simulink model "dualFisheyeSim"  (R2024b)
settings: Solver=VariableStepAuto  StartTime=0.0  StopTime=10.0  RelTol=1e-3
undefined symbols (not defined in the file): Sim3dSensor
libraries: sim3dcameralib x2, sim3dautolib x1, sim3dlib x1, visionsinks x1
settings Model: Creator=cuixingxing  LastModifiedBy=Administrator
settings ModelReferenceCC: EnableRefExpFcnMdlSchedulingChecks=on
settings RTWCC: GPUComputeCapability=3.5

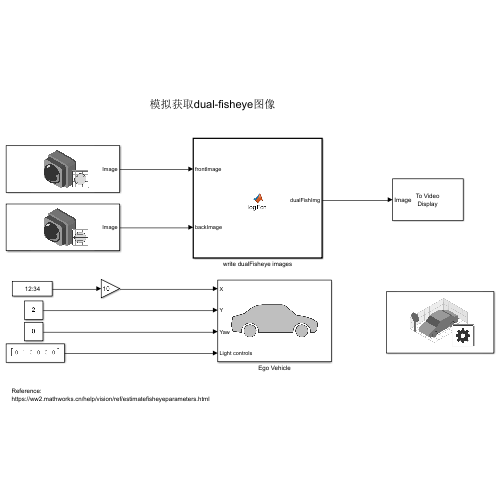
[thumbnail: Simulink's stored preview of the top-level diagram]
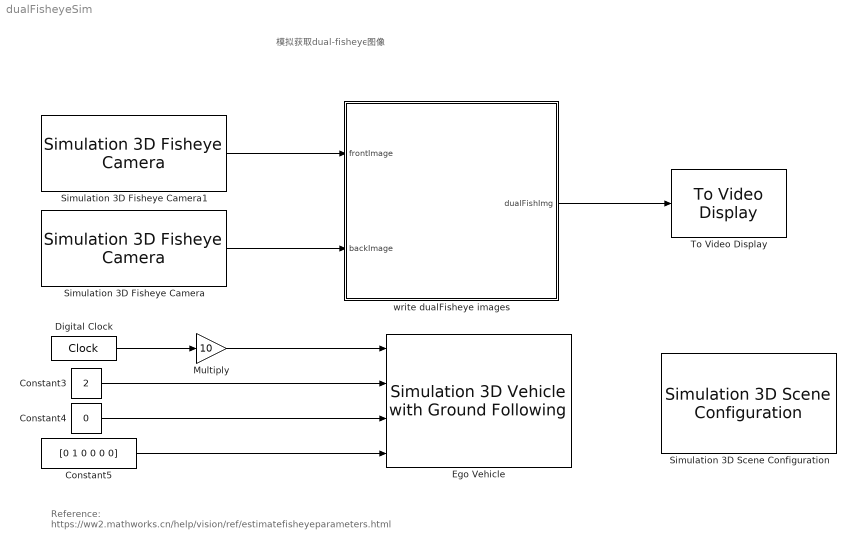
== system dualFisheyeSim ==
  note: Reference:
      | https://ww2.mathworks.cn/help/vision/ref/estimatefisheyeparameters.html
  note: 模拟获取dual-fisheye图像
  Constant3 : Constant  Value=2
  Constant4 : Constant  Value=0
  Constant5 : Constant  Value=[0 1 0 0 0 0]
  Digital Clock : DigitalClock  SampleTime=0.01
  Ego Vehicle : sim3dautolib/Simulation 3D Vehicle with Ground Following  Priority=-1  PassVehMesh=Hatchback  MeshPath=/MathWorksSimulation/Vehicles/Muscle/Meshes/SK_MuscleCar.SK_MuscleCar  TrackWidth=1.9  WheelBase=3  WheelRadius=0.35  VehColor=Red  InitialPos=[45, 0, 0]  InitialRot=[0, 0, 90]  ActorName=SimulinkVehicle  SampleTime=-1  ActorType=SimulinkVehicle  ID=C  aMode=3  ActorTag=SimulinkVehicle  CoordinateScheme=ISO  VehLightsControl=on  HeadlightColor=[ 1, 1, 1 ]  HighBeamIntensity=100000  LowBeamIntensity=60000  HighBeamConeAngle=70  LowBeamConeAngle=70  LeftHeadlightOrientation=[ 0, 0 ]  RightHeadlightOrientation=[ 0, 0 ]  BrakelightIntensity=500  ReverselightIntensity=500  SignallightIntensity=500  SignallightPeriod=1  SignalPulseWidth=50  TransformOutportEnabled=off
      settings: LibrarySourceBlock=drivingsim3d/Simulation 3D Vehicle with Ground Following
  Multiply : Gain  Gain=10
  Simulation 3D Fisheye Camera : sim3dcameralib/Simulation 3D Fisheye Camera  Priority=1  sensorTag=Sim3dSensor�  sensorId=1  sensorName=Sim3dSensor�  vehTagList={'Scene Origin';'SimulinkVehicle'}  vehTag=SimulinkVehicle  mountLoc=Origin  offsetFlag=on  tmountOffset=[0, 0, 2.5]  extTmount=off  rmountOffset=[0, 0, 0]  extRmount=off  OpticalCenter=[376,376]  ImageSize=[752,752]  RadialDistortion=[235.8351 -0.0024 6.9258e-06 -1.6209e-08]  StretchMatrix=[1, 0; 0, 1]  TransformOutportEnabled=off  SampleTime=-1  mountPoint=[0 0 2.5]  mountOrientation=[0 0 0]  aMode=3  ID=1
      settings: LibrarySourceBlock=drivingsim3d/Simulation 3D Fisheye Camera
  Simulation 3D Fisheye Camera1 : sim3dcameralib/Simulation 3D Fisheye Camera  Priority=1  sensorTag=Sim3dSensor�  sensorId=2  sensorName=Sim3dSensor�  vehTagList={'Scene Origin';'SimulinkVehicle'}  vehTag=SimulinkVehicle  mountLoc=Origin  offsetFlag=on  tmountOffset=[0, 0, 2.5]  extTmount=off  rmountOffset=[0, 0, 180]  extRmount=off  OpticalCenter=[376,376]  ImageSize=[752,752]  RadialDistortion=[235.8351 -0.0024 6.9258e-06 -1.6209e-08]  StretchMatrix=[1, 0; 0, 1]  TransformOutportEnabled=off  SampleTime=-1  mountPoint=[0 0 2.5]  mountOrientation=[0 0 -180]  aMode=3  ID=2
      settings: LibrarySourceBlock=drivingsim3d/Simulation 3D Fisheye Camera
  Simulation 3D Scene Configuration : sim3dlib/Simulation 3D Scene Configuration  Priority=0  ProjectFormat=Default Scenes  SceneDesc=US city block  ProjectName=C:\Program Files\MATLAB\R2024b\toolbox\shared\sim3d_projects\automotive_project_windows\UE\WindowsNoEditor\VehicleSimulation.exe  ScenePath=/Game/Maps/HwStrght  EnableOpenDRIVE=off  vehTagList={'Scene Origin';'SimulinkVehicle'}  vehTag=Scene Origin  FreeCameraInitialTranslation=[0, 0, 0]  FreeCameraDefaultInitialTranslation=[-6, 0, 2]  FreeCameraInitialRotation=[0, 0, 0]  FreeCameraDefaultInitialRotation=[0, -15, 0]  OpVisEn=off  Ts=1/60  EnableWindow=on  EnableRemoteAccess=off  EnableWeather=off  SunAzimuth=90  SunAltitude=40.0  EnableGeospatialSun=off  Latitude=0  Longitude=0  Date=2023-01-01  Time=10:30:00  GeoTimeZone=-5.0  SunDaylightSaving=off  wind=1  clouds=10  EnableVolumetricClouds=off  CloudCoverage=0  CloudAltitude=6  fog=0  rain=0  RaindropsEffect=off  SnowDensity=0  EnableGeospatial=off  UseTrueOrigin=off  OriginHeight=200  OriginLatitude=40.744652  OriginLongitude=-73.988864  MapStyle=Aerial  AdditionalAssetIDs=[]  UseAdvancedSunSky=off  SolarTime=11  TimeZone=-5  Day=21  Month=9  Year=2022  UseDaylightSavingTime=on  DSTStartDay=10  DSTStartMonth=3  DSTEndDay=3  DSTEndMonth=11  DSTSwitchHour=2  sensorTag=MainCamera1  sensorId=1  sensorName=MainCamera1  mountLoc=Origin  offsetFlag=off  tmountOffset=[0, 0, 0]  rmountOffset=[0, 0, 0]  HorizontalResolution=1280  VerticalResolution=720  HorizontalFOV=60  mountPoint=[0 0 0]  mountOrientation=[0 0 0]  aMode=3  ID=1  GeoTrigger=Inactive
      settings: LibrarySourceBlock=drivingsim3d/Simulation 3D Scene Configuration
  To Video Display : visionsinks/To Video Display  windowSizeMode=Normal  openAtMdlStart=on  fullScreen=off  videoWindowX=653  videoWindowY=203  saveWindowSize=off  videoWindowWidth=1504  videoWindowHeight=752  inputColorFormat=RGB  inputType=Obsolete  imagePorts=One multidimensional signal  OutputDevice=On-screen video monitor  dataOrg=Column-major  isWindowOpen=off
  write dualFisheye images : MATLAB Function  TreatAsAtomicUnit=on
  wires:
  Simulation 3D Fisheye Camera/1 -> write dualFisheye images/2(backImage)
  Constant4/1 -> Ego Vehicle/3
  Multiply/1 -> Ego Vehicle/1
  Digital Clock/1 -> Multiply/1
  Constant5/1 -> Ego Vehicle/4
  Constant3/1 -> Ego Vehicle/2
  Simulation 3D Fisheye Camera1/1 -> write dualFisheye images/1(frontImage)
  write dualFisheye images/1(dualFishImg) -> To Video Display/1

== matlab function dualFisheyeSim/write dualFisheye images ==
  data: frontImage input; backImage input; dualFishImg output
function dualFishImg = logFcn(frontImage,backImage)

arguments
    frontImage
    backImage
end
coder.extrinsic("sprintf","imwrite","insertShape");

% step1: initialize variables 
persistent numStep maskImgRGB
if isempty(numStep)
    numStep = 1;
    [h,w,c] = size(frontImage);
    maskImgRGB = zeros([h,w,c],"like",frontImage);
    maskImgRGB = insertShape(maskImgRGB,"filled-circle",[w/2,h/2,h/2],ShapeColor="white",Opacity = 1);
end


% step2: write current images
img1Name = sprintf("./%05d.jpg",numStep);

mask = logical(maskImgRGB);

f1 = maskImgRGB;
f2 = maskImgRGB;
f1(mask) = frontImage(mask);
f2(mask) = backImage(mask);
dualFishImg = [f1,f2];
imwrite(dualFishImg,img1Name);

% step3: numStep plus one
numStep  = numStep+1;
end
